simulink model "Simulador_Lazaro_Preanalisis"  (R2025b)
settings: Solver=ode45  StartTime=0.0  StopTime=6  RelTol=1e-3  EnableMultiTasking=on
libraries: slpidlib x1
settings Model: Creator=Administrador  LastModifiedBy=richards
settings SolverCC: ZeroCrossControl=DisableAll  AlgebraicLoopSolver=TrustRegion
settings DataIOCC: LimitDataPoints=on  SaveFormat=Array  SignalLoggingSaveFormat=ModelDataLogs  ReturnWorkspaceOutputs=off
settings OptimizationCC: ExpressionDepthLimit=2147483647.0  LifeSpan=inf
settings DebuggingCC: UnderspecifiedInitializationDetection=Classic  MergeDetectMultiDrivingBlocksExec=none  SolverPrmCheckMsg=warning  FcnCallInpInsideContextMsg=warning  UnconnectedInputMsg=warning  UnconnectedOutputMsg=warning  UnconnectedLineMsg=warning  StateNameClashWarn=warning  SFUnexpectedBacktrackingDiag=warning  SFNoUnconditionalDefaultTransitionDiag=warning  SFExecutionAtInitializationDiag=none  ArithmeticOperatorsInVariantConditions=warning
settings HardwareCC: ProdBitPerPointer=32.0  ProdBitPerSizeT=32.0  ProdBitPerPtrDiffT=32.0  ProdLargestAtomicFloat=None  ProdIntDivRoundTo=Undefined  ProdEndianess=Unspecified  ProdWordSize=32.0  ProdHWDeviceType=32-bit Generic
settings ModelReferenceCC: EnableRefExpFcnMdlSchedulingChecks=on  PropagateSignalLabelsOutOfModel=off
settings SFSimCC: SimUseLocalCustomCode=off  SimParseCustomCode=off  CustomCodeUndefinedFunction=UseInterfaceOnly
settings RTWCC: RTWUseLocalCustomCode=off  GPUComputeCapability=3.5
settings CodeAppCC: StateflowObjectComments=on
settings GRTTargetCC: TargetLangStandard=C89/C90 (ANSI)  CombineOutputUpdateFcns=off  GRTInterface=on
settings ConfigComp: CovMetricSettings=dw  CovSaveCumulativeToWorkspaceVar=on  CovSaveSingleToWorkspaceVar=on  CovExternalEMLEnable=off

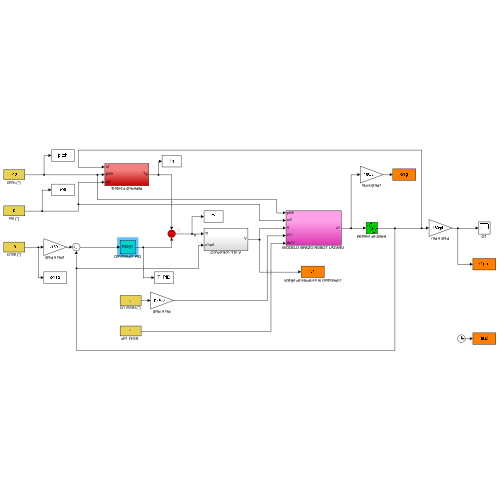
[thumbnail: Simulink's stored preview of the top-level diagram]
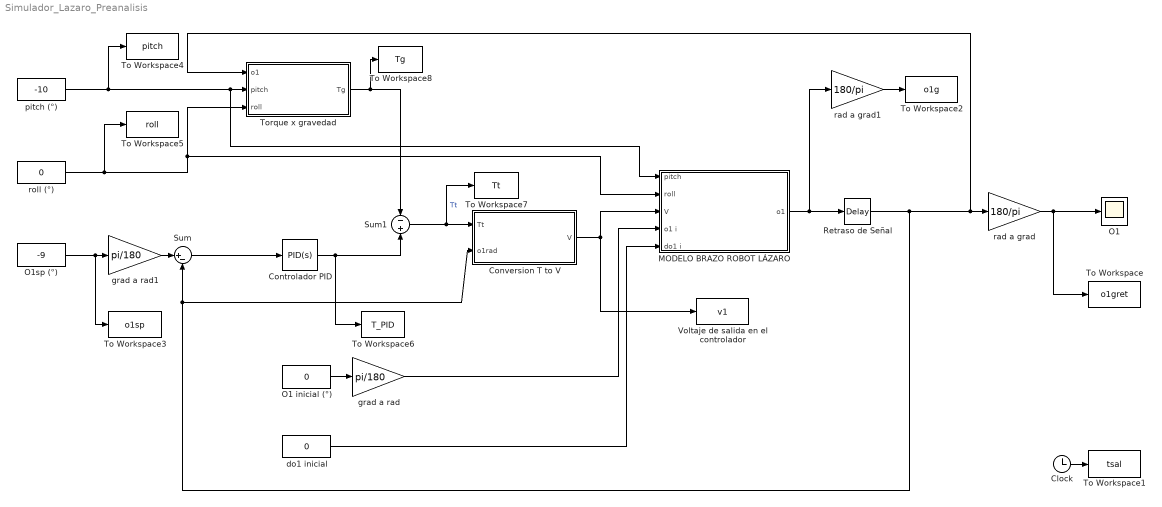
== system Simulador_Lazaro_Preanalisis ==
  Clock : Clock
  Controlador PID : slpidlib/PID Controller  Controller=PID  Form=Parallel  TimeDomain=Continuous-time  UseExternalTs=off  SampleTime=1  IntegratorMethod=Forward Euler  FilterMethod=Forward Euler  ControllerParametersSource=internal  P=5  I=0.2  UseKiTs=off  D=2  UseExternalDerivativeSource=off  N=100  UseFilter=on  TunerSelectOption=Transfer Function Based (PID Tuner App)  InitialConditionSource=internal  InitialConditionForIntegrator=0  InitialConditionForFilter=0  DifferentiatorICPrevScaledInput=0  ExternalReset=none  TrackingMode=off  Kt=1  LimitOutput=off  SatLimitsSource=internal  UpperSaturationLimit=inf  LowerSaturationLimit=-inf  LinearizeAsGain=off  AntiWindupMode=none  Kb=1  LimitIntegrator=off  UpperIntegratorSaturationLimit=inf  LowerIntegratorSaturationLimit=-inf  POutMin=[]  POutMax=[]  IOutMin=[]  IOutMax=[]  DOutMin=[]  DOutMax=[]  NOutMin=[]  NOutMax=[]  SumOutMin=[]  SumOutMax=[]  SaturationOutMin=[]  SaturationOutMax=[]  PParamMin=[]  PParamMax=[]  IParamMin=[]  IParamMax=[]  DParamMin=[]  DParamMax=[]  NParamMin=[]  NParamMax=[]  KbParamMin=[]  KbParamMax=[]  KtParamMin=[]  KtParamMax=[]  KbOutMin=[]  KbOutMax=[]  KtOutMin=[]  KtOutMax=[]  IntegratorOutMin=[]  IntegratorOutMax=[]  FilterOutMin=[]  FilterOutMax=[]  SumI1OutMin=[]  SumI1OutMax=[]  SumI2OutMin=[]  SumI2OutMax=[]  SumI3OutMin=[]  SumI3OutMax=[]  SumI4OutMin=[]  SumI4OutMax=[]  SumDOutMin=[]  SumDOutMax=[]  DifferentiatorOutMin=[]  DifferentiatorOutMax=[]  FilterDiffOutCoefMin=[]  FilterDiffOutCoefMax=[]  ReciprocalOutMin=[]  ReciprocalOutMax=[]  SumDenOutMin=[]  SumDenOutMax=[]  SumNumOutMin=[]  SumNumOutMax=[]  DivideOutMin=[]  DivideOutMax=[]  UdiffTsProdOutMin=[]  UdiffTsProdOutMax=[]  NTsProdOutMin=[]  NTsProdOutMax=[]  UintegralTsProdOutMin=[]  UintegralTsProdOutMax=[]  UngainTsProdOutMin=[]  UngainTsProdOutMax=[]  ClampingZeroOutDataTypeStr=Inherit: Inherit via back propagation  ClampingZeroOutMin=[]  ClampingZeroOutMax=[]  FilterDenConstantOutDataTypeStr=Inherit: Inherit via back propagation  FilterDenConstantOutMin=[]  FilterDenConstantOutMax=[]  PCopyOutDataTypeStr=Inherit: Inherit via back propagation  PCopyOutMin=[]  PCopyOutMax=[]  NCopyOutDataTypeStr=Inherit: Inherit via back propagation  NCopyOutMin=[]  NCopyOutMax=[]  IntegratorContinuousStateAttributes=''  IntegratorStateMustResolveToSignalObject=off  IntegratorRTWStateStorageClass=Auto  FilterContinuousStateAttributes=''  FilterStateMustResolveToSignalObject=off  FilterRTWStateStorageClass=Auto  ParallelPVariant=InternalParameters  IdealPVariant=Disabled  IVariant=InternalParameters  DVariant=InternalParameters  IntegratorVariant=Continuous  SatVariant=Disabled  AWVariant=Passthrough  PCopyVariant=Disabled  TRVariant=Disabled  FdbkBlocksVariant=Forward  IdealPFdbkVariant=Disabled  SatFdbkVariant=Disabled  DerivativeFilterVariant=ContFilter  NVariant=InternalParameters  NCopyVariant=Disabled  FilterICVariant=InternalICsFilter  IntegratorICVariant=InternalICs  ExternalResetVariant=Disabled  TRSumVariant=Passthrough  SumFdbkVariant=Disabled  SumVariant=Sum_PID  TsampFilterVariant=InternalTs  TsampNgainVariant=Passthrough  TsampIntegralVariant=Disabled_SignalSpec  ExternalSaturationOutDataTypeStr=Inherit: Same as second input  DerivativeSourceVariant=ErrorSignal  PreIntVariant=InternalPreInt
  Conversion T to V : Subsystem
  MODELO BRAZO ROBOT LÁZARO : Subsystem
  O1 : Scope
      settings: TimeSpan=20  ActiveDisplayYMinimum=-1  ActiveDisplayYMaximum=1  DataLoggingMaxPoints=50000
  O1 inicial (°) : Constant  Value=0
  O1sp (°) : Constant  Value=-9  OutDataTypeStr=Inherit: Inherit via back propagation
  Retraso de Señal : TransportDelay  DelayTime=0
  Sum : Sum  Inputs=|+-
  Sum1 : Sum  Inputs=-+
  To Workspace : ToWorkspace  VariableName=o1gret  SampleTime=-1
  To Workspace1 : ToWorkspace  VariableName=tsal  SampleTime=-1
  To Workspace2 : ToWorkspace  VariableName=o1g  SampleTime=-1
  To Workspace3 : ToWorkspace  VariableName=o1sp  SampleTime=-1
  To Workspace4 : ToWorkspace  VariableName=pitch  SampleTime=-1
  To Workspace5 : ToWorkspace  VariableName=roll  SampleTime=-1
  To Workspace6 : ToWorkspace  VariableName=T_PID  SampleTime=-1
  To Workspace7 : ToWorkspace  VariableName=Tt  SampleTime=-1
  To Workspace8 : ToWorkspace  VariableName=Tg  SampleTime=-1
  Torque x gravedad : Subsystem
  Voltaje de salida en el controlador : ToWorkspace  VariableName=v1  SampleTime=-1
  "do1 inicial " : Constant  Value=0
  grad a rad : Gain  Gain=pi/180
  grad a rad1 : Gain  Gain=pi/180
  pitch (°) : Constant  Value=-10
  rad a grad : Gain  Gain=180/pi
  rad a grad1 : Gain  Gain=180/pi
  roll (°) : Constant  Value=0
  wires:
  O1 inicial (°)/1 -> grad a rad/1
  rad a grad/1 -> To Workspace/1, O1/1
  grad a rad1/1 -> Sum/1
  Sum/1 -> Controlador PID/1
  MODELO BRAZO ROBOT LÁZARO/1(o1) -> rad a grad1/1, Retraso de Señal/1
  grad a rad/1 -> MODELO BRAZO ROBOT LÁZARO/4(o1 i)
  "do1 inicial "/1 -> MODELO BRAZO ROBOT LÁZARO/5(do1 i)
  Clock/1 -> To Workspace1/1
  rad a grad1/1 -> To Workspace2/1
  Conversion T to V/1(V) -> MODELO BRAZO ROBOT LÁZARO/3(V), Voltaje de salida en el controlador/1
  Controlador PID/1 -> To Workspace6/1, Sum1/2
  Sum1/1 -> To Workspace7/1, Conversion T to V/1(Tt)  "Tt"
  Retraso de Señal/1 -> rad a grad/1, Torque x gravedad/1(o1), Conversion T to V/2(o1rad), Sum/2
  roll (°)/1 -> Torque x gravedad/3(roll), MODELO BRAZO ROBOT LÁZARO/2(roll), To Workspace5/1
  O1sp (°)/1 -> grad a rad1/1, To Workspace3/1
  pitch (°)/1 -> Torque x gravedad/2(pitch), MODELO BRAZO ROBOT LÁZARO/1(pitch), To Workspace4/1
  Torque x gravedad/1(Tg) -> Sum1/1, To Workspace8/1

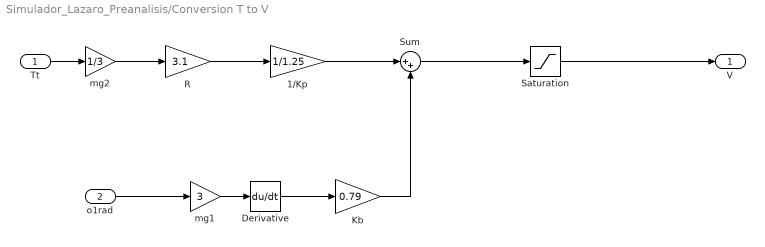
== system Simulador_Lazaro_Preanalisis/Conversion T to V ==
  Tt : Inport
  o1rad : Inport  Port=2
  1/Kp : Gain  Gain=1/1.25
  Derivative : Derivative
  Kb : Gain  Gain=0.79
  R : Gain  Gain=3.1
  Saturation : Saturate  UpperLimit=6  LowerLimit=-6
  Sum : Sum  Inputs=|++
  mg1 : Gain  Gain=3
  mg2 : Gain  Gain=1/3
  V : Outport
  wires:
  o1rad/1 -> mg1/1
  mg1/1 -> Derivative/1
  Derivative/1 -> Kb/1
  Tt/1 -> mg2/1
  R/1 -> 1/Kp/1
  1/Kp/1 -> Sum/1
  Kb/1 -> Sum/2
  Sum/1 -> Saturation/1
  mg2/1 -> R/1
  Saturation/1 -> V/1

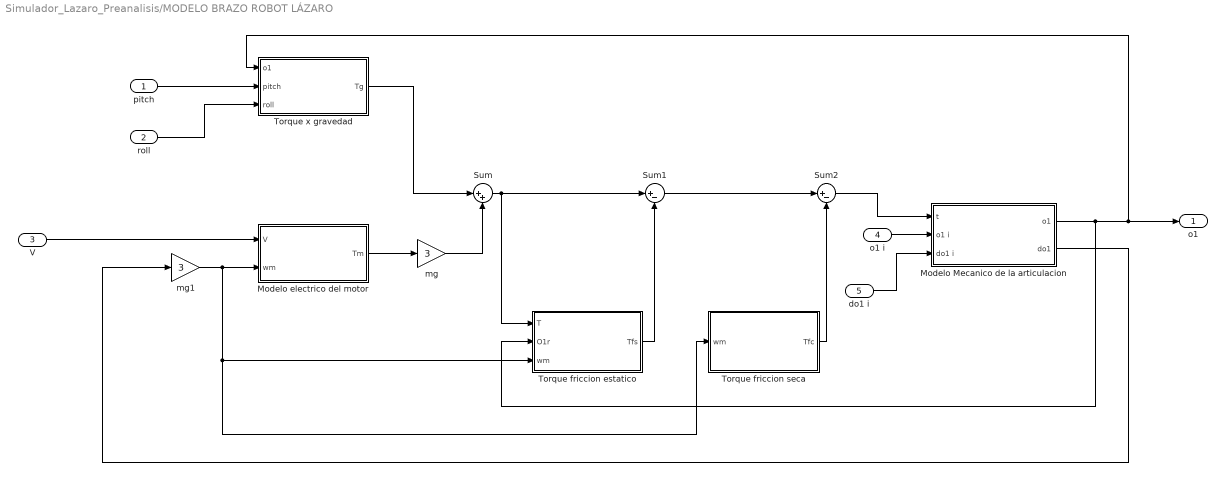
== system Simulador_Lazaro_Preanalisis/MODELO BRAZO ROBOT LÁZARO ==
  pitch : Inport
  roll : Inport  Port=2
  V : Inport  Port=3
  o1 i : Inport  Port=4
  do1 i : Inport  Port=5
  Modelo Mecanico de la articulacion : Subsystem
  Modelo electrico del motor : Subsystem
  Sum : Sum  Inputs=|++
  Sum1 : Sum  Inputs=|+-
  Sum2 : Sum  Inputs=|+-
  Torque friccion estatico : Subsystem
  Torque friccion seca : Subsystem
  Torque x gravedad : Subsystem
  mg : Gain  Gain=3
  mg1 : Gain  Gain=3
  o1 : Outport
  wires:
  pitch/1 -> Torque x gravedad/2(pitch)
  roll/1 -> Torque x gravedad/3(roll)
  Modelo Mecanico de la articulacion/1(o1) -> o1/1, Torque x gravedad/1(o1), Torque friccion estatico/2(O1r)
  Sum/1 -> Sum1/1, Torque friccion estatico/1(T)
  Torque x gravedad/1(Tg) -> Sum/1
  Modelo electrico del motor/1(Tm) -> mg/1
  Modelo Mecanico de la articulacion/2(do1) -> mg1/1
  V/1 -> Modelo electrico del motor/1(V)
  mg1/1 -> Modelo electrico del motor/2(wm), Torque friccion estatico/3(wm), Torque friccion seca/1(wm)
  o1 i/1 -> Modelo Mecanico de la articulacion/2(o1 i)
  do1 i/1 -> Modelo Mecanico de la articulacion/3(do1 i)
  Sum1/1 -> Sum2/1
  Sum2/1 -> Modelo Mecanico de la articulacion/1(t)
  Torque friccion estatico/1(Tfs) -> Sum1/2
  Torque friccion seca/1(Tfc) -> Sum2/2
  mg/1 -> Sum/2

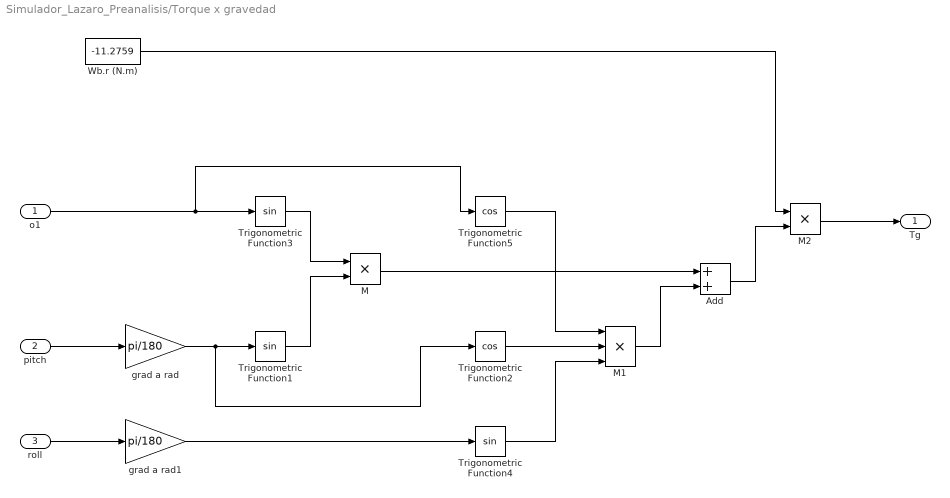
== system Simulador_Lazaro_Preanalisis/Torque x gravedad ==
  o1 : Inport
  pitch : Inport  Port=2
  roll : Inport  Port=3
  Add : Sum
  M : Product  Inputs=**
  M1 : Product  Inputs=***
  M2 : Product  Inputs=**
  Trigonometric Function1 : Trigonometry
  Trigonometric Function2 : Trigonometry  Operator=cos
  Trigonometric Function3 : Trigonometry
  Trigonometric Function4 : Trigonometry
  Trigonometric Function5 : Trigonometry  Operator=cos
  Wb.r (N.m) : Constant  Value=-11.2759
  grad a rad : Gain  Gain=pi/180
  grad a rad1 : Gain  Gain=pi/180
  Tg : Outport
  wires:
  pitch/1 -> grad a rad/1
  grad a rad/1 -> Trigonometric Function1/1, Trigonometric Function2/1
  o1/1 -> Trigonometric Function3/1, Trigonometric Function5/1
  Trigonometric Function1/1 -> M/2
  Trigonometric Function3/1 -> M/1
  Trigonometric Function2/1 -> M1/2
  Trigonometric Function4/1 -> M1/3
  Trigonometric Function5/1 -> M1/1
  M/1 -> Add/1
  M1/1 -> Add/2
  Add/1 -> M2/2
  Wb.r (N.m)/1 -> M2/1
  M2/1 -> Tg/1
  roll/1 -> grad a rad1/1
  grad a rad1/1 -> Trigonometric Function4/1

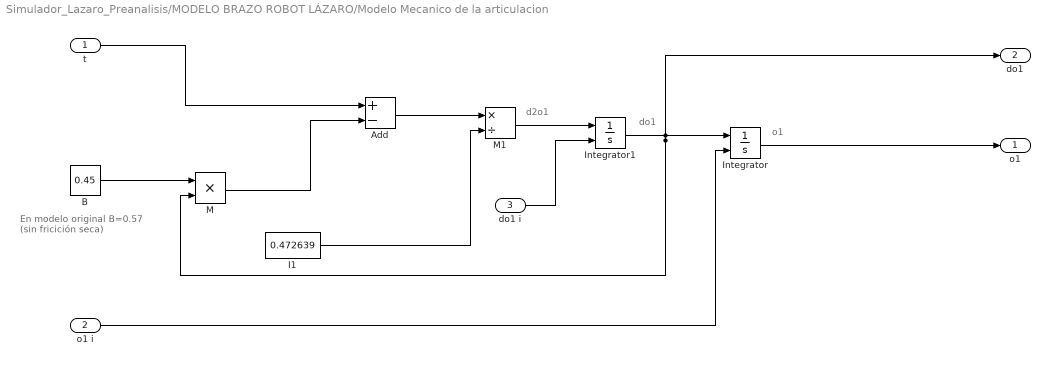
== system Simulador_Lazaro_Preanalisis/MODELO BRAZO ROBOT LÁZARO/Modelo Mecanico de la articulacion ==
  note: o1
  note: d2o1
  note: do1
  note: En modelo original B=0.57
      | (sin fricición seca)
  t : Inport
  o1 i : Inport  Port=2
  do1 i : Inport  Port=3
  Add : Sum  Inputs=+-
  B : Constant  Value=0.45
  I1 : Constant  Value=0.472639
  Integrator : Integrator  InitialConditionSource=external
  Integrator1 : Integrator  InitialConditionSource=external
  M : Product  Inputs=**
  M1 : Product  Inputs=*/
  o1 : Outport
  do1 : Outport  Port=2
  wires:
  Integrator/1 -> o1/1
  t/1 -> Add/1
  B/1 -> M/1
  M/1 -> Add/2
  Add/1 -> M1/1
  I1/1 -> M1/2
  M1/1 -> Integrator1/1
  Integrator1/1 -> M/2, Integrator/1, do1/1
  o1 i/1 -> Integrator/2
  do1 i/1 -> Integrator1/2

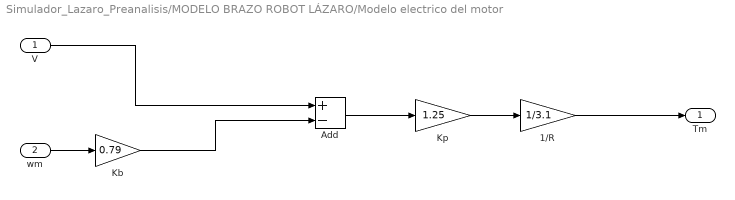
== system Simulador_Lazaro_Preanalisis/MODELO BRAZO ROBOT LÁZARO/Modelo electrico del motor ==
  V : Inport
  wm : Inport  Port=2
  1/R : Gain  Gain=1/3.1
  Add : Sum  Inputs=+-
  Kb : Gain  Gain=0.79
  Kp : Gain  Gain=1.25
  Tm : Outport
  wires:
  V/1 -> Add/1
  Add/1 -> Kp/1
  Kp/1 -> 1/R/1
  1/R/1 -> Tm/1
  wm/1 -> Kb/1
  Kb/1 -> Add/2

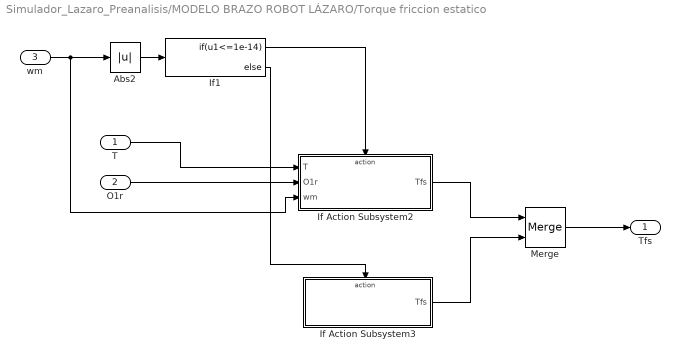
== system Simulador_Lazaro_Preanalisis/MODELO BRAZO ROBOT LÁZARO/Torque friccion estatico ==
  T : Inport
  O1r : Inport  Port=2
  wm : Inport  Port=3
  Abs2 : Abs  SaturateOnIntegerOverflow=off
  If Action Subsystem2 : Subsystem  TreatAsAtomicUnit=on
  If Action Subsystem3 : Subsystem  TreatAsAtomicUnit=on
  If1 : If  IfExpression=u1<=1e-14
  Merge : Merge
  Tfs : Outport
  wires:
  Abs2/1 -> If1/1
  wm/1 -> Abs2/1, If Action Subsystem2/3(wm)
  T/1 -> If Action Subsystem2/1(T)
  O1r/1 -> If Action Subsystem2/2(O1r)
  If1/1 -> If Action Subsystem2/Action
  If1/2 -> If Action Subsystem3/Action
  If Action Subsystem2/1(Tfs) -> Merge/1
  If Action Subsystem3/1(Tfs) -> Merge/2
  Merge/1 -> Tfs/1

== system Simulador_Lazaro_Preanalisis/MODELO BRAZO ROBOT LÁZARO/Torque friccion seca ==
  wm : Inport
  Abs2 : Abs  SaturateOnIntegerOverflow=off
  If Action Subsystem2 : Subsystem  TreatAsAtomicUnit=on
  If Action Subsystem3 : Subsystem  TreatAsAtomicUnit=on
  If1 : If  IfExpression=u1>1e-14
  Merge : Merge
  Tfc : Outport
  wires:
  Abs2/1 -> If1/1
  wm/1 -> Abs2/1, If Action Subsystem2/1(wm)
  If1/1 -> If Action Subsystem2/Action
  If1/2 -> If Action Subsystem3/Action
  If Action Subsystem2/1(Tfc) -> Merge/1
  If Action Subsystem3/1(Tfc) -> Merge/2
  Merge/1 -> Tfc/1

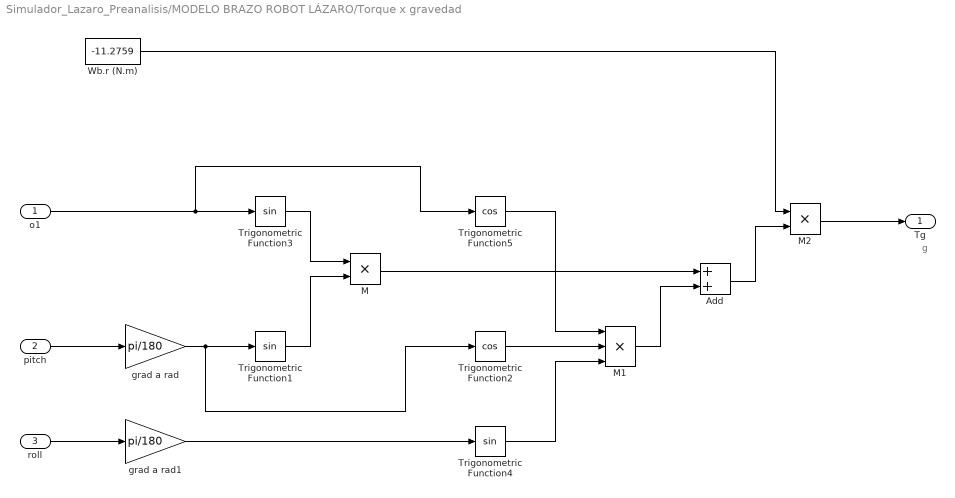
== system Simulador_Lazaro_Preanalisis/MODELO BRAZO ROBOT LÁZARO/Torque x gravedad ==
  note: g
  o1 : Inport
  pitch : Inport  Port=2
  roll : Inport  Port=3
  Add : Sum
  M : Product  Inputs=**
  M1 : Product  Inputs=***
  M2 : Product  Inputs=**
  Trigonometric Function1 : Trigonometry
  Trigonometric Function2 : Trigonometry  Operator=cos
  Trigonometric Function3 : Trigonometry
  Trigonometric Function4 : Trigonometry
  Trigonometric Function5 : Trigonometry  Operator=cos
  Wb.r (N.m) : Constant  Value=-11.2759
  grad a rad : Gain  Gain=pi/180
  grad a rad1 : Gain  Gain=pi/180
  Tg : Outport
  wires:
  pitch/1 -> grad a rad/1
  grad a rad/1 -> Trigonometric Function1/1, Trigonometric Function2/1
  o1/1 -> Trigonometric Function3/1, Trigonometric Function5/1
  Trigonometric Function1/1 -> M/2
  Trigonometric Function3/1 -> M/1
  Trigonometric Function2/1 -> M1/2
  Trigonometric Function4/1 -> M1/3
  Trigonometric Function5/1 -> M1/1
  M/1 -> Add/1
  M1/1 -> Add/2
  Add/1 -> M2/2
  Wb.r (N.m)/1 -> M2/1
  M2/1 -> Tg/1
  roll/1 -> grad a rad1/1
  grad a rad1/1 -> Trigonometric Function4/1

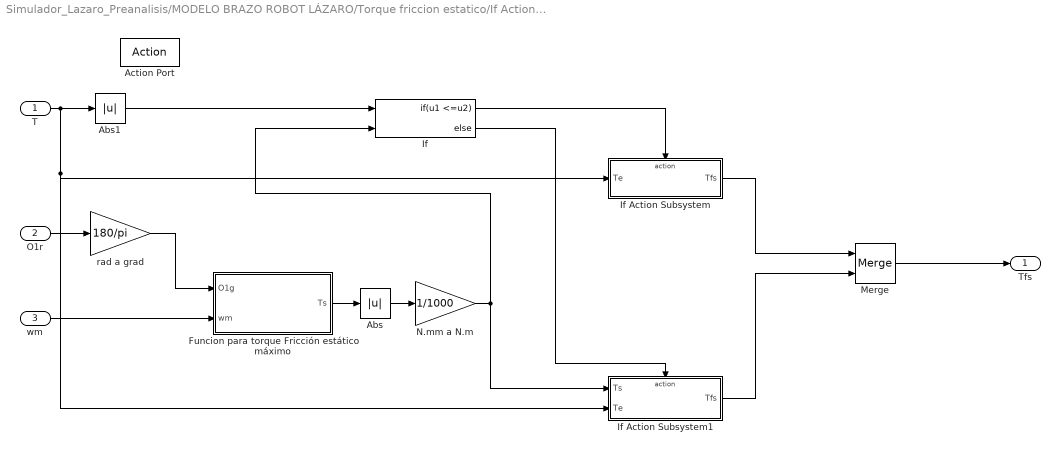
== system Simulador_Lazaro_Preanalisis/MODELO BRAZO ROBOT LÁZARO/Torque friccion estatico/If Action Subsystem2 ==
  T : Inport
  O1r : Inport  Port=2
  wm : Inport  Port=3
  Action Port : ActionPort  ActionPortLabel=if(u1<=1e-14)
  Abs : Abs  SaturateOnIntegerOverflow=off
  Abs1 : Abs  SaturateOnIntegerOverflow=off
  Funcion para torque Fricción estático máximo : Subsystem
  If : If  NumInputs=2  IfExpression=u1 <=u2
  If Action Subsystem : Subsystem  TreatAsAtomicUnit=on
  If Action Subsystem1 : Subsystem  TreatAsAtomicUnit=on
  Merge : Merge
  N.mm a N.m : Gain  Gain=1/1000
  rad a grad : Gain  Gain=180/pi
  Tfs : Outport
  wires:
  O1r/1 -> rad a grad/1
  rad a grad/1 -> Funcion para torque Fricción estático máximo/1(O1g)
  wm/1 -> Funcion para torque Fricción estático máximo/2(wm)
  Funcion para torque Fricción estático máximo/1(Ts) -> Abs/1
  T/1 -> Abs1/1, If Action Subsystem1/2(Te), If Action Subsystem/1(Te)
  Abs1/1 -> If/1
  Abs/1 -> N.mm a N.m/1
  If/1 -> If Action Subsystem/Action
  If/2 -> If Action Subsystem1/Action
  If Action Subsystem/1(Tfs) -> Merge/1
  If Action Subsystem1/1(Tfs) -> Merge/2
  N.mm a N.m/1 -> If/2, If Action Subsystem1/1(Ts)
  Merge/1 -> Tfs/1

== system Simulador_Lazaro_Preanalisis/MODELO BRAZO ROBOT LÁZARO/Torque friccion estatico/If Action Subsystem3 ==
  Action Port : ActionPort  ActionPortLabel=else
  Constant : Constant  Value=0
  Tfs : Outport
  wires:
  Constant/1 -> Tfs/1

== system Simulador_Lazaro_Preanalisis/MODELO BRAZO ROBOT LÁZARO/Torque friccion seca/If Action Subsystem2 ==
  wm : Inport
  Action Port : ActionPort  ActionPortLabel=if(u1>1e-14)
  Constant : Constant  Value=0.3
  Product : Product  RndMeth=Zero
  Sign : Signum
  Tfc : Outport
  wires:
  wm/1 -> Sign/1
  Sign/1 -> Product/1
  Constant/1 -> Product/2
  Product/1 -> Tfc/1

== system Simulador_Lazaro_Preanalisis/MODELO BRAZO ROBOT LÁZARO/Torque friccion seca/If Action Subsystem3 ==
  Action Port : ActionPort  ActionPortLabel=else
  Constant : Constant  Value=0
  Tfc : Outport
  wires:
  Constant/1 -> Tfc/1

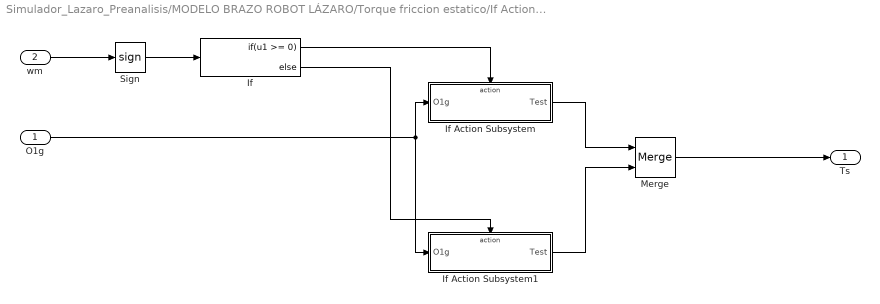
== system Simulador_Lazaro_Preanalisis/MODELO BRAZO ROBOT LÁZARO/Torque friccion estatico/If Action Subsystem2/Funcion para torque Fricción estático máximo ==
  O1g : Inport
  wm : Inport  Port=2
  If : If  IfExpression=u1 >= 0
  If Action Subsystem : Subsystem  TreatAsAtomicUnit=on
  If Action Subsystem1 : Subsystem  TreatAsAtomicUnit=on
  Merge : Merge
  Sign : Signum
  Ts : Outport
  wires:
  wm/1 -> Sign/1
  Sign/1 -> If/1
  If/1 -> If Action Subsystem/Action
  If/2 -> If Action Subsystem1/Action
  If Action Subsystem/1(Test) -> Merge/1
  If Action Subsystem1/1(Test) -> Merge/2
  Merge/1 -> Ts/1
  O1g/1 -> If Action Subsystem/1(O1g), If Action Subsystem1/1(O1g)

== system Simulador_Lazaro_Preanalisis/MODELO BRAZO ROBOT LÁZARO/Torque friccion estatico/If Action Subsystem2/If Action Subsystem ==
  Te : Inport
  Action Port : ActionPort  ActionPortLabel=if(u1 <=u2)
  Tfs : Outport
  wires:
  Te/1 -> Tfs/1

== system Simulador_Lazaro_Preanalisis/MODELO BRAZO ROBOT LÁZARO/Torque friccion estatico/If Action Subsystem2/If Action Subsystem1 ==
  Ts : Inport
  Te : Inport  Port=2
  Action Port : ActionPort  ActionPortLabel=else
  Product : Product  RndMeth=Zero
  Sign : Signum
  Tfs : Outport
  wires:
  Ts/1 -> Product/1
  Product/1 -> Tfs/1
  Te/1 -> Sign/1
  Sign/1 -> Product/2

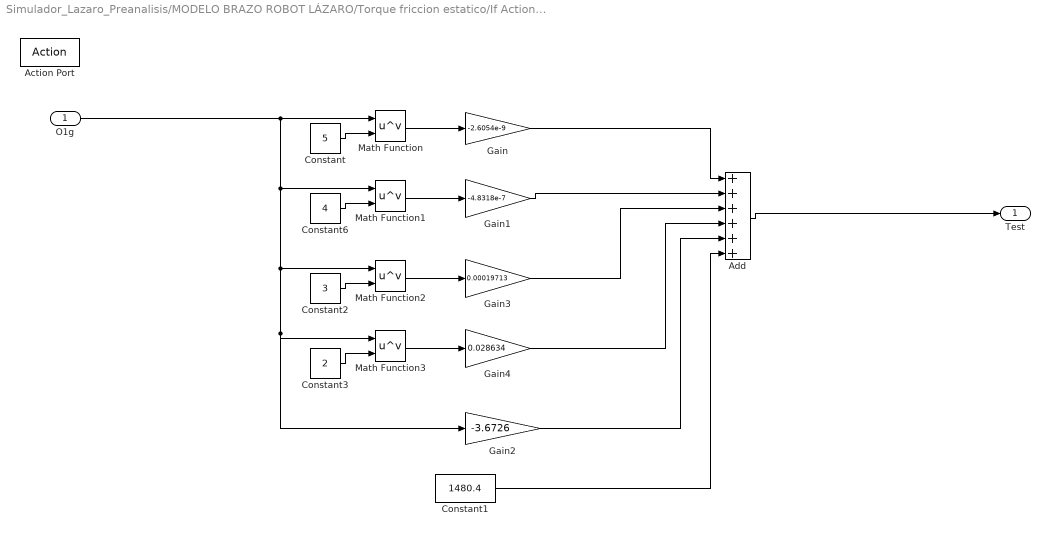
== system Simulador_Lazaro_Preanalisis/MODELO BRAZO ROBOT LÁZARO/Torque friccion estatico/If Action Subsystem2/Funcion para torque Fricción estático máximo/If Action Subsystem ==
  O1g : Inport
  Action Port : ActionPort  ActionPortLabel=if(u1 >= 0)
  Add : Sum  Inputs=++++++
  Constant : Constant  Value=5
  Constant1 : Constant  Value=1480.4
  Constant2 : Constant  Value=3
  Constant3 : Constant  Value=2
  Constant6 : Constant  Value=4
  Gain : Gain  Gain=-2.6054e-9
  Gain1 : Gain  Gain=-4.8318e-7
  Gain2 : Gain  Gain=-3.6726
  Gain3 : Gain  Gain=0.00019713
  Gain4 : Gain  Gain=0.028634
  Math Function{,1..3} (4 alike) : Math  Operator=pow  SignedPower=on
  Test : Outport
  wires:
  Add/1 -> Test/1
  Constant/1 -> Math Function/2
  Constant6/1 -> Math Function1/2
  Gain/1 -> Add/1
  Gain1/1 -> Add/2
  Math Function/1 -> Gain/1
  Math Function1/1 -> Gain1/1
  O1g/1 -> Math Function/1, Math Function1/1, Math Function2/1, Math Function3/1, Gain2/1
  Constant2/1 -> Math Function2/2
  Math Function2/1 -> Gain3/1
  Constant3/1 -> Math Function3/2
  Math Function3/1 -> Gain4/1
  Gain4/1 -> Add/4
  Gain3/1 -> Add/3
  Gain2/1 -> Add/5
  Constant1/1 -> Add/6

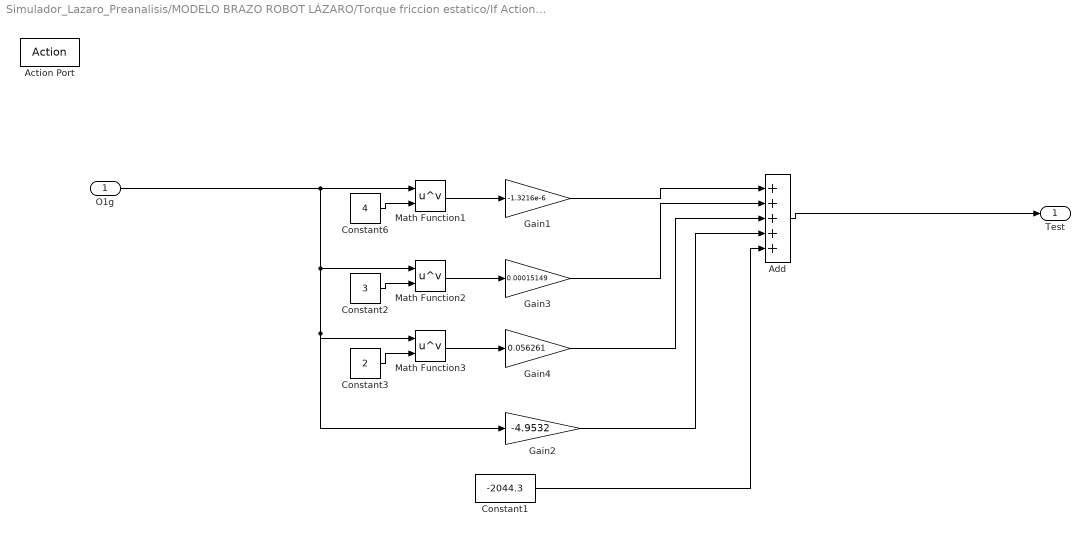
== system Simulador_Lazaro_Preanalisis/MODELO BRAZO ROBOT LÁZARO/Torque friccion estatico/If Action Subsystem2/Funcion para torque Fricción estático máximo/If Action Subsystem1 ==
  O1g : Inport
  Action Port : ActionPort  ActionPortLabel=else
  Add : Sum  Inputs=+++++
  Constant1 : Constant  Value=-2044.3
  Constant2 : Constant  Value=3
  Constant3 : Constant  Value=2
  Constant6 : Constant  Value=4
  Gain1 : Gain  Gain=-1.3216e-6
  Gain2 : Gain  Gain=-4.9532
  Gain3 : Gain  Gain=0.00015149
  Gain4 : Gain  Gain=0.056261
  Math Function1 : Math  Operator=pow  SignedPower=on
  Math Function2 : Math  Operator=pow  SignedPower=on
  Math Function3 : Math  Operator=pow  SignedPower=on
  Test : Outport
  wires:
  Add/1 -> Test/1
  Constant6/1 -> Math Function1/2
  Math Function1/1 -> Gain1/1
  O1g/1 -> Math Function1/1, Math Function2/1, Math Function3/1, Gain2/1
  Constant2/1 -> Math Function2/2
  Math Function2/1 -> Gain3/1
  Constant3/1 -> Math Function3/2
  Math Function3/1 -> Gain4/1
  Constant1/1 -> Add/5
  Gain1/1 -> Add/1
  Gain3/1 -> Add/2
  Gain4/1 -> Add/3
  Gain2/1 -> Add/4
